simulink model "PRE6"  (R2021a)
settings: Solver=ode23t  StartTime=0.0  StopTime=0.01  MaxStep=1e-6  RelTol=1e-3
settings Model: Creator=Dell  LastModifiedBy=Dell

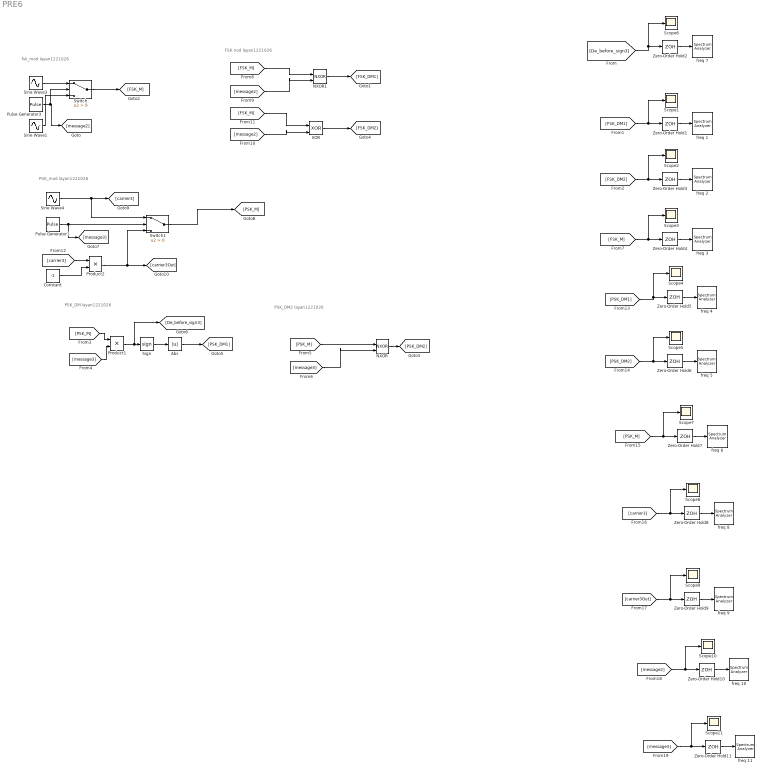
== system PRE6 ==
  note: FSK nod layan1221026
  note: fsk_mod layan1221026
  note: PSK_DM layan1221026
  note: PSK_DM2 layan1221026
  note: PSK_mod layan1221026
   freq {1..11} (11 alike) : SpectrumAnalyzer
  Abs : Abs
  Constant : Constant  Value=-1
  NXOR : Logic  Operator=NXOR  IconShape=distinctive  AllPortsSameDT=off  OutDataTypeStr=boolean
  NXOR1 : Logic  Operator=NXOR  IconShape=distinctive  AllPortsSameDT=off  OutDataTypeStr=boolean
  Product1 : Product
  Product2 : Product
  Pulse Generator1 : DiscretePulseGenerator  PulseType=Time based  Period=0.002  PulseWidth=50
  Pulse Generator3 : DiscretePulseGenerator  PulseType=Time based  Period=0.002  PulseWidth=50
  Scope{1..11} (11 alike) : Scope
  Sign : Signum
  Sine Wave1 : Sin  Frequency=2*pi*25000  Samples=5  SampleTime=1e-6
  Sine Wave3 : Sin  Frequency=2*pi*15000  Samples=5  SampleTime=1e-6
  Sine Wave4 : Sin  Frequency=2*pi*20000  Samples=5  SampleTime=1e-6
  Switch : Switch  Criteria=u2 > Threshold
  Switch1 : Switch  Criteria=u2 > Threshold
  XOR : Logic  Operator=XOR  IconShape=distinctive  AllPortsSameDT=off  OutDataTypeStr=boolean
  Zero-Order Hold{1..11} (11 alike) : ZeroOrderHold  SampleTime=-1
  wires:
  Pulse Generator3/1 -> Switch/2, [message2]
  [PSK_M] -> Product1/1
  [message3] -> Product1/2
  Product1/1 -> [De_before_sign3], Sign/1
  Sign/1 -> Abs/1
  Abs/1 -> [PSK_DM1]
  NXOR/1 -> [PSK_DM2]
  [PSK_M] -> NXOR/1
  [message3] -> NXOR/2
  Sine Wave3/1 -> Switch/1
  Sine Wave1/1 -> Switch/3
  Switch/1 -> [FSK_M]
  [FSK_M] -> NXOR1/1
  [FSK_M] -> XOR/1
  [message2] -> NXOR1/2
  NXOR1/1 -> [FSK_DM1]
  [message2] -> XOR/2
  XOR/1 -> [FSK_DM2]
  Sine Wave4/1 -> [carrier3], Switch1/1
  Pulse Generator1/1 -> Switch1/2, [message3]
  Switch1/1 -> [PSK_M]
  [carrier3] -> Product2/1
  Constant/1 -> Product2/2
  Product2/1 -> [carrier3Out], Switch1/3
  Zero-Order Hold2/1 -> " freq 7"/1
  [De_before_sign3] -> Scope6/1, Zero-Order Hold2/1
  Zero-Order Hold1/1 -> " freq 1"/1
  [FSK_DM1] -> Scope1/1, Zero-Order Hold1/1
  Zero-Order Hold3/1 -> " freq 2"/1
  [FSK_DM2] -> Scope2/1, Zero-Order Hold3/1
  Zero-Order Hold4/1 -> " freq 3"/1
  [FSK_M] -> Scope3/1, Zero-Order Hold4/1
  Zero-Order Hold5/1 -> " freq 4"/1
  [PSK_DM1] -> Scope4/1, Zero-Order Hold5/1
  Zero-Order Hold6/1 -> " freq 5"/1
  [PSK_DM2] -> Scope5/1, Zero-Order Hold6/1
  [PSK_M] -> Scope7/1, Zero-Order Hold7/1
  Zero-Order Hold7/1 -> " freq 6"/1
  [carrier3] -> Scope8/1, Zero-Order Hold8/1
  Zero-Order Hold8/1 -> " freq 8"/1
  [carrier3Out] -> Scope9/1, Zero-Order Hold9/1
  Zero-Order Hold9/1 -> " freq 9"/1
  [message2] -> Scope10/1, Zero-Order Hold10/1
  Zero-Order Hold10/1 -> " freq 10"/1
  Zero-Order Hold11/1 -> " freq 11"/1
  [message3] -> Scope11/1, Zero-Order Hold11/1
